simulink model "bai2222"  (R2018a)
settings: Solver=ode4  StartTime=0.0  StopTime=60  FixedStep=0.01  RelTol=1e-3
libraries: fuzblock x1
settings Model: Creator=ADMIN  LastModifiedBy=ADMIN

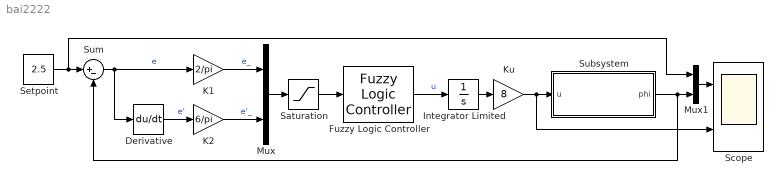
== system bai2222 ==
  Derivative : Derivative
  Fuzzy Logic Controller : fuzblock/Fuzzy Logic  Controller  FIS='BDK2.fis'  OutputSampleNumber=101  DataType=double  FuzzifiedInputs=off  RuleFiringStrengths=off  RuleOutputs=off  AggregatedOutputs=off  SimulateUsing=Interpreted execution  OutOfRangeInputValueMessage=warning  NoRuleFiredMessage=warning  EmptyOutputFuzzySetMessage=warning
  Integrator Limited : Integrator  LimitOutput=on  UpperSaturationLimit=1  LowerSaturationLimit=0
  K1 : Gain  Gain=2/pi
  K2 : Gain  Gain=6/pi
  Ku : Gain  Gain=8
  Mux : Mux  Inputs=2
  Mux1 : Mux  Inputs=2
  Saturation : Saturate  UpperLimit=1  LowerLimit=-1
  Scope : Scope  NumInputPorts=2
  "Setpoint " : Constant  Value=2.5
  Subsystem : Subsystem  mask{J=0.05, M=1, m_=0.1, l=4, lc=0.15, B=0.2, g=9.81, phi0=0, phidot0=0}
      mask prompts: J "moment quan tinh"; M "Khoi luong canh tay may"; m_ "Khoi luong vat nang"; l "Chieu dai canh tay may"; lc "Khoang cac tu trong tam den truc quay"; B "He so ma sat nhot"; g "Gia toc trong truong"; phi0 "Goc quay ban dau"; phidot0 "Van toc goc ban dau"
  Sum : Sum  Inputs=|+-
  wires:
  Mux1/1 -> Scope/1
  Saturation/1 -> Fuzzy Logic Controller/1
  K2/1 -> Mux/2  "e'_"
  Mux/1 -> Saturation/1
  K1/1 -> Mux/1  "e_"
  "Setpoint "/1 -> Mux1/1, Sum/1
  Subsystem/1("phi ") -> Mux1/2, Sum/2
  Derivative/1 -> K2/1  "e'"
  Sum/1 -> K1/1, Derivative/1  "e"
  Fuzzy Logic Controller/1 -> Integrator Limited/1  "u"
  Integrator Limited/1 -> Ku/1
  Ku/1 -> Scope/2, Subsystem/1("u ")

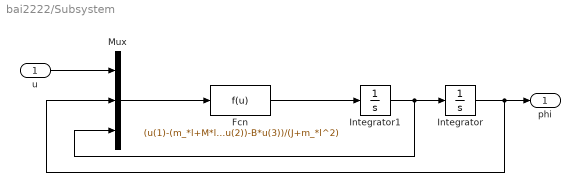
== system bai2222/Subsystem ==
  "u " : Inport
  Fcn : Fcn  Expr=(u(1)-(m_*l+M*lc)*g*sin(u(2))-B*u(3))/(J+m_*l^2)
  Integrator : Integrator  InitialCondition=phi0
  Integrator1 : Integrator  InitialCondition=phidot0
  Mux : Mux  Inputs=3
  "phi " : Outport
  wires:
  Integrator/1 -> Mux/2, "phi "/1
  Integrator1/1 -> Mux/3, Integrator/1
  "u "/1 -> Mux/1
  Mux/1 -> Fcn/1
  Fcn/1 -> Integrator1/1
